simulink model "CaseD"  (R2016b)
settings: Solver=FixedStepAuto  StartTime=0.0  StopTime=time  FixedStep=dt  RelTol=1e-3
values from neighbouring files (symbols this model uses):
  C = [6; 0]    [main.m]
  dt = 0.01    [main.m]
  initial_eta = [1 0 0]'    [main.m]
  initial_eta_2 = [6 5 0]'    [main.m]
  initial_eta_4 = [7 0 0]'    [main.m]
  K_p = diag([0.2,0.2,0.1])    [main.m]
  mu = 0.1    [main.m]
  P_d = [2  0 ... (first row only)    [main.m]
  R = diag(r)    [main.m]
  r = [5; 3]    [main.m]
  U_max = 1    [main.m]
  U_ref = [(0:dt:time)' [zeros(floor(1*points/6),1) ... (first row only)    [main.m]
libraries: simulink x1
(part 1 of 2)
settings Model: Creator=helene  LastModifiedBy=kefin

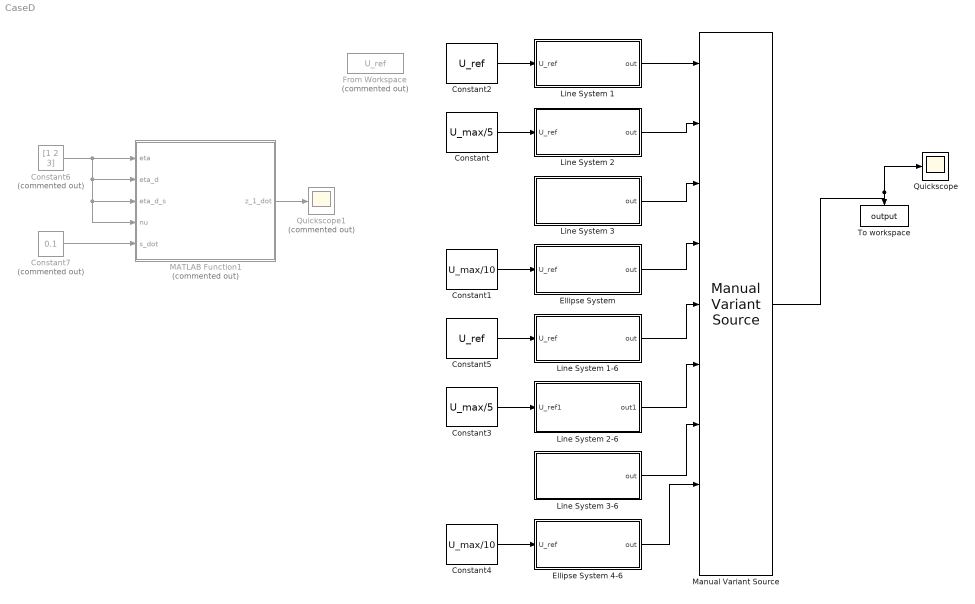
== system CaseD ==
  Constant : Constant  Value=U_max/5
  Constant1 : Constant  Value=U_max/10
  Constant2 : Constant  Value=U_ref
  Constant3 : Constant  Value=U_max/5
  Constant4 : Constant  Value=U_max/10
  Constant5 : Constant  Value=U_ref
  Constant6 : Constant  Commented=on  Value=[1 2 3]
  Constant7 : Constant  Commented=on  Value=0.1
  Ellipse System : Subsystem
  Ellipse System 4-6 : Subsystem
  From Workspace : FromWorkspace  Commented=on  VariableName=U_ref  SampleTime=dt
  Line System 1 : Subsystem
  Line System 1-6 : Subsystem
  Line System 2 : Subsystem
  Line System 2-6 : Subsystem
  Line System 3 : Subsystem
  Line System 3-6 : Subsystem
  MATLAB Function1 : MATLAB Function  Commented=on  TreatAsAtomicUnit=on
  Manual Variant Source : simulink/Signal Routing/Manual Variant Source  NumChoices=9  OverrideUsingVariant=V_8
  Quickscope : Scope
  Quickscope1 : Scope  Commented=on
  To workspace : ToWorkspace  VariableName=output  SampleTime=-1
      settings: StopFcn=plotting
  wires:
  Ellipse System/1(out) -> Manual Variant Source/4
  Manual Variant Source/1 -> Quickscope/1, To workspace/1
  Line System 1/1(out) -> Manual Variant Source/1
  Line System 2/1(out) -> Manual Variant Source/2
  Constant/1 -> Line System 2/1(U_ref)
  Line System 3/1(out) -> Manual Variant Source/3
  Constant1/1 -> Ellipse System/1(U_ref)
  Constant2/1 -> Line System 1/1(U_ref)
  Ellipse System 4-6/1(out) -> Manual Variant Source/8
  Line System 1-6/1(out) -> Manual Variant Source/5
  Line System 2-6/1(out1) -> Manual Variant Source/6
  Constant3/1 -> Line System 2-6/1(U_ref1)
  Line System 3-6/1(out) -> Manual Variant Source/7
  Constant4/1 -> Ellipse System 4-6/1(U_ref)
  Constant5/1 -> Line System 1-6/1(U_ref)
  Constant6/1 -> MATLAB Function1/4(nu), MATLAB Function1/3(eta_d_s), MATLAB Function1/2(eta_d), MATLAB Function1/1(eta)
  Constant7/1 -> MATLAB Function1/5(s_dot)
  MATLAB Function1/1(z_1_dot) -> Quickscope1/1

== system CaseD/Ellipse System ==
  U_ref : Inport
  Control law : Subsystem
  "Ellipse Mapper " : Subsystem
  Ellipse Speed Gauge : Subsystem
  Kinematic model : Subsystem
  Mux : Mux  Inputs=3
  Update Law : Subsystem
  out : Outport
  wires:
  U_ref/1 -> Ellipse Speed Gauge/1(U_ref)
  Update Law/1(s) -> Mux/3, Ellipse Speed Gauge/2(s), "Ellipse Mapper "/1(s)
  "Ellipse Mapper "/1(eta_d) -> Update Law/2(eta_d), Mux/2, Control law/4(eta_d)
  Kinematic model/1("eta ") -> Control law/1(eta), Update Law/4(eta), Mux/1
  Control law/1(nu) -> Kinematic model/1(nu)
  "Ellipse Mapper "/2(eta_d_s) -> Control law/3(eta_d_s), Update Law/3(eta_d_s)
  Ellipse Speed Gauge/1(U_s) -> Control law/2(U_s), Update Law/1(U_s)
  Mux/1 -> out/1

== system CaseD/Ellipse System 4-6 ==
  U_ref : Inport
  Control law1 : Subsystem
  "Ellipse Mapper " : Subsystem
  Ellipse Speed Gauge : Subsystem
  Kinematic model : Subsystem
  Mux : Mux  Inputs=3
  Update Law : Subsystem
  out : Outport
  wires:
  U_ref/1 -> Ellipse Speed Gauge/1(U_ref)
  Update Law/1(s) -> Ellipse Speed Gauge/2(s), "Ellipse Mapper "/1(s), Mux/3
  "Ellipse Mapper "/1(eta_d) -> Control law1/3(eta_d), Update Law/2(eta_d), Mux/2
  Kinematic model/1("eta ") -> Control law1/7(eta), Update Law/4(eta), Mux/1
  Control law1/1(new_nu) -> Control law1/8(nu), Kinematic model/1(nu)
  "Ellipse Mapper "/2(eta_d_s) -> Update Law/3(eta_d_s), Control law1/2(eta_d_s)
  Ellipse Speed Gauge/1(U_s) -> Control law1/1(U_s), Update Law/1(U_s)
  Mux/1 -> out/1
  Update Law/2(s_dot) -> Control law1/4(s_dot)
  Ellipse Speed Gauge/2(U_s_s) -> Control law1/5(U_s_s)
  "Ellipse Mapper "/3(eta_d_ss) -> Control law1/6(eta_d_ss)

== system CaseD/Line System 1 ==
  U_ref : Inport
  Control law : Subsystem
  Kinematic model : Subsystem
  Line Mapper : Subsystem
  Line Speed Gauge : Subsystem
  Mux : Mux  Inputs=3
  Update Law : Subsystem
  out : Outport
  wires:
  U_ref/1 -> Line Speed Gauge/1(U_ref)
  Update Law/1(s) -> Mux/3, Line Mapper/1("s ")
  Control law/1(nu) -> Kinematic model/1(nu)
  Line Mapper/2(eta_d_s) -> Control law/3(eta_d_s), Update Law/3(eta_d_s)
  Line Speed Gauge/1(U_s) -> Control law/2(U_s), Update Law/1(U_s)
  Line Mapper/1(eta_d) -> Control law/4(eta_d), Update Law/2(eta_d), Mux/2
  Kinematic model/1("eta ") -> Control law/1(eta), Update Law/4(eta), Mux/1
  Mux/1 -> out/1

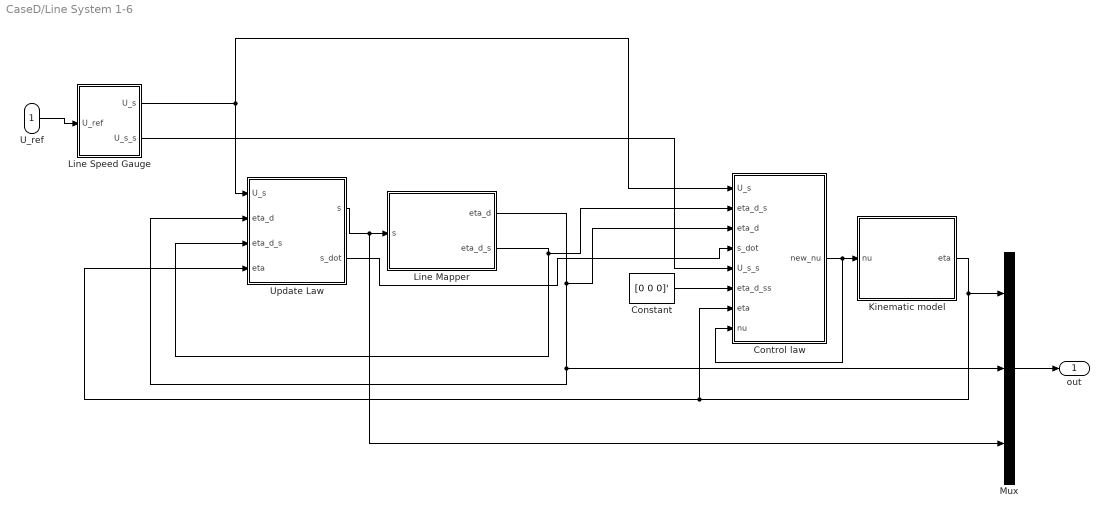
== system CaseD/Line System 1-6 ==
  U_ref : Inport
  Constant : Constant  Value=[0 0 0]'
  Control law : Subsystem
  Kinematic model : Subsystem
  Line Mapper : Subsystem
  Line Speed Gauge : Subsystem
  Mux : Mux  Inputs=3
  Update Law : Subsystem
  out : Outport
  wires:
  U_ref/1 -> Line Speed Gauge/1(U_ref)
  Update Law/1(s) -> Mux/3, Line Mapper/1("s ")
  Control law/1(new_nu) -> Control law/8(nu), Kinematic model/1(nu)
  Line Mapper/2(eta_d_s) -> Control law/2(eta_d_s), Update Law/3(eta_d_s)
  Line Speed Gauge/1(U_s) -> Control law/1(U_s), Update Law/1(U_s)
  Line Mapper/1(eta_d) -> Control law/3(eta_d), Update Law/2(eta_d), Mux/2
  Kinematic model/1("eta ") -> Control law/7(eta), Update Law/4(eta), Mux/1
  Mux/1 -> out/1
  Update Law/2(s_dot) -> Control law/4(s_dot)
  Line Speed Gauge/2(U_s_s) -> Control law/5(U_s_s)
  Constant/1 -> Control law/6(eta_d_ss)

== system CaseD/Line System 2 ==
  U_ref : Inport
  Control law : Subsystem
  Kinematic model : Subsystem
  Line Mapper : Subsystem
  Line Speed Gauge : Subsystem
  Mux : Mux  Inputs=3
  Update Law : Subsystem
  out : Outport
  wires:
  U_ref/1 -> Line Speed Gauge/1(U_ref)
  Update Law/1(s) -> Mux/3, Line Mapper/1("s ")
  Control law/1(nu) -> Kinematic model/1(nu)
  Line Mapper/2(eta_d_s) -> Update Law/3(eta_d_s), Control law/3(eta_d_s)
  Line Speed Gauge/1(U_s) -> Control law/2(U_s), Update Law/1(U_s)
  Line Mapper/1(eta_d) -> Update Law/2(eta_d), Mux/2, Control law/4(eta_d)
  Kinematic model/1("eta ") -> Control law/1(eta), Update Law/4(eta), Mux/1
  Mux/1 -> out/1

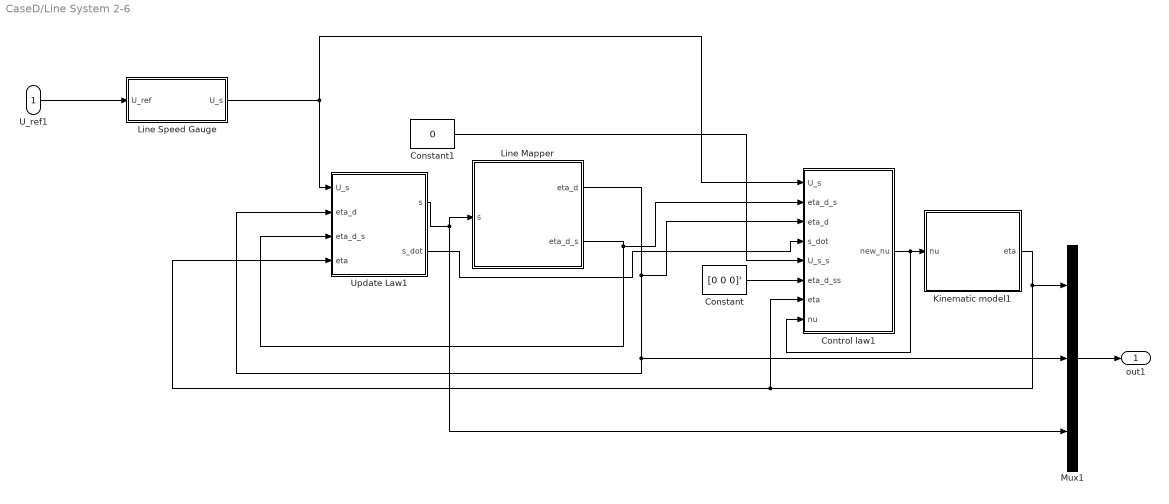
== system CaseD/Line System 2-6 ==
  U_ref1 : Inport
  Constant : Constant  Value=[0 0 0]'
  Constant1 : Constant  Value=0
  Control law1 : Subsystem
  Kinematic model1 : Subsystem
  Line Mapper : Subsystem
  Line Speed Gauge : Subsystem
  Mux1 : Mux  Inputs=3
  Update Law1 : Subsystem
  out1 : Outport
  wires:
  U_ref1/1 -> Line Speed Gauge/1(U_ref)
  Update Law1/1(s) -> Line Mapper/1("s "), Mux1/3
  Control law1/1(new_nu) -> Control law1/8(nu), Kinematic model1/1(nu)
  Line Mapper/2(eta_d_s) -> Control law1/2(eta_d_s), Update Law1/3(eta_d_s)
  Line Speed Gauge/1(U_s) -> Control law1/1(U_s), Update Law1/1(U_s)
  Line Mapper/1(eta_d) -> Control law1/3(eta_d), Update Law1/2(eta_d), Mux1/2
  Kinematic model1/1("eta ") -> Control law1/7(eta), Update Law1/4(eta), Mux1/1
  Mux1/1 -> out1/1
  Update Law1/2(s_dot) -> Control law1/4(s_dot)
  Constant1/1 -> Control law1/5(U_s_s)
  Constant/1 -> Control law1/6(eta_d_ss)

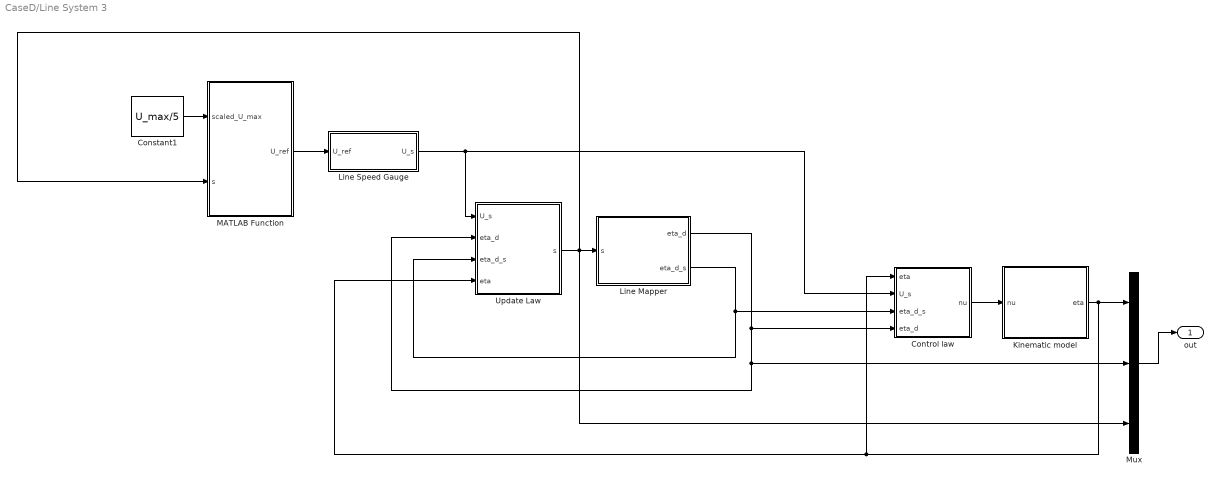
== system CaseD/Line System 3 ==
  Constant1 : Constant  Value=U_max/5
  Control law : Subsystem
  Kinematic model : Subsystem
  Line Mapper : Subsystem
  Line Speed Gauge : Subsystem
  MATLAB Function : MATLAB Function  TreatAsAtomicUnit=on
  Mux : Mux  Inputs=3
  Update Law : Subsystem
  out : Outport
  wires:
  Update Law/1(s) -> Line Mapper/1(s), Mux/3, MATLAB Function/2(s)
  Control law/1(nu) -> Kinematic model/1(nu)
  Line Mapper/2(eta_d_s) -> Control law/3(eta_d_s), Update Law/3(eta_d_s)
  Line Speed Gauge/1(U_s) -> Control law/2(U_s), Update Law/1(U_s)
  Line Mapper/1(eta_d) -> Control law/4(eta_d), Update Law/2(eta_d), Mux/2
  Kinematic model/1("eta ") -> Control law/1(eta), Update Law/4(eta), Mux/1
  Mux/1 -> out/1
  MATLAB Function/1(U_ref) -> Line Speed Gauge/1(U_ref)
  Constant1/1 -> MATLAB Function/1(scaled_U_max)

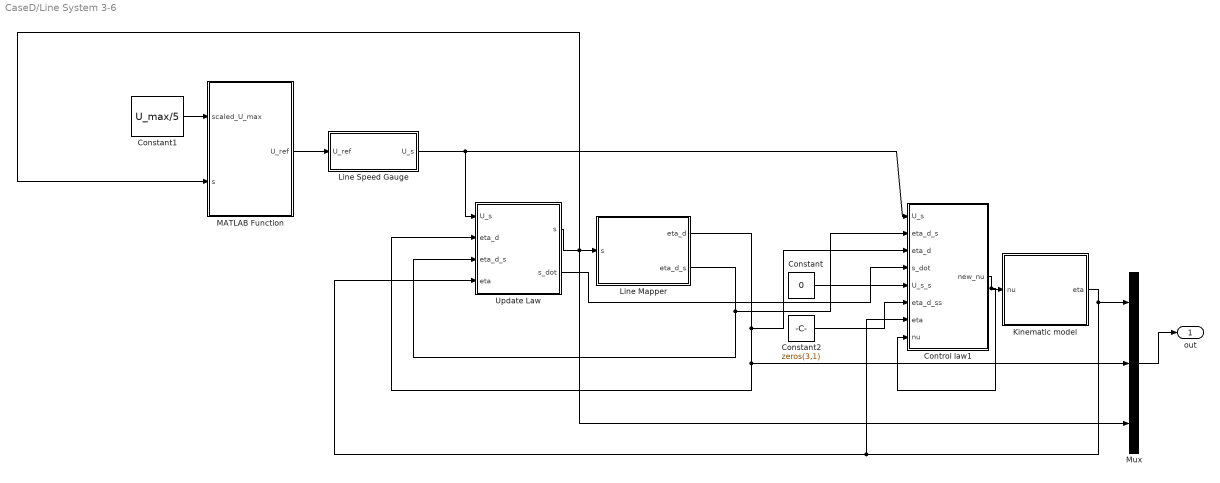
== system CaseD/Line System 3-6 ==
  Constant : Constant  Value=0
  Constant1 : Constant  Value=U_max/5
  Constant2 : Constant  Value=zeros(3,1)
  Control law1 : Subsystem
  Kinematic model : Subsystem
  Line Mapper : Subsystem
  Line Speed Gauge : Subsystem
  MATLAB Function : MATLAB Function  TreatAsAtomicUnit=on
  Mux : Mux  Inputs=3
  Update Law : Subsystem
  out : Outport
  wires:
  Update Law/1(s) -> Line Mapper/1(s), Mux/3, MATLAB Function/2(s)
  Control law1/1(new_nu) -> Control law1/8(nu), Kinematic model/1(nu)
  Line Mapper/2(eta_d_s) -> Control law1/2(eta_d_s), Update Law/3(eta_d_s)
  Line Speed Gauge/1(U_s) -> Control law1/1(U_s), Update Law/1(U_s)
  Line Mapper/1(eta_d) -> Control law1/3(eta_d), Update Law/2(eta_d), Mux/2
  Kinematic model/1("eta ") -> Control law1/7(eta), Update Law/4(eta), Mux/1
  Mux/1 -> out/1
  MATLAB Function/1(U_ref) -> Line Speed Gauge/1(U_ref)
  Constant1/1 -> MATLAB Function/1(scaled_U_max)
  Update Law/2(s_dot) -> Control law1/4(s_dot)
  Constant/1 -> Control law1/5(U_s_s)
  Constant2/1 -> Control law1/6(eta_d_ss)

== system CaseD/Ellipse System/Control law ==
  eta : Inport
  U_s : Inport  Port=2
  eta_d_s : Inport  Port=3
  eta_d : Inport  Port=4
  Control Law : MATLAB Function  TreatAsAtomicUnit=on
  K_p : Constant  Value=K_p
  Scope : Scope
  nu : Outport
  wires:
  K_p/1 -> Control Law/1(K_p)
  Control Law/1(nu) -> nu/1
  eta_d_s/1 -> Control Law/4(eta_d_s)
  U_s/1 -> Control Law/5(U_s)
  eta_d/1 -> Control Law/3(eta_d)
  eta/1 -> Control Law/2(eta)
  Control Law/2(z_1) -> Scope/1

== system CaseD/Ellipse System/Ellipse Mapper  ==
  s : Inport
  Constant : Constant  Value=R
  Constant1 : Constant  Value=C
  Ellipse Mapper : MATLAB Function  TreatAsAtomicUnit=on
  eta_d : Outport  PortDimensions=3
  eta_d_s : Outport  Port=2  PortDimensions=3
  wires:
  Ellipse Mapper/1(eta_d) -> eta_d/1
  Ellipse Mapper/2(eta_d_s) -> eta_d_s/1
  Constant1/1 -> Ellipse Mapper/2(C)
  Constant/1 -> Ellipse Mapper/3(R)
  s/1 -> Ellipse Mapper/1(s)

== system CaseD/Ellipse System/Ellipse Speed Gauge ==
  U_ref : Inport
  s : Inport  Port=2
  Constant : Constant  Value=r
  Ellipse : MATLAB Function  TreatAsAtomicUnit=on
  U_s : Outport
  wires:
  U_ref/1 -> Ellipse/1(U_ref)
  Ellipse/1(U_s) -> U_s/1
  Constant/1 -> Ellipse/3(r)
  s/1 -> Ellipse/2(s)

== system CaseD/Ellipse System/Kinematic model ==
  nu : Inport
  Integrator : Integrator  InitialCondition=initial_eta_4
  MATLAB Function : MATLAB Function  TreatAsAtomicUnit=on
  Product : Product  Multiplication=Matrix(*)
  Rotation matrix : MATLAB Function  TreatAsAtomicUnit=on
  Selector : Selector  InputPortWidth=3  IndexOptions=Starting index (dialog)  Indices=3  OutputSizes=1
  "eta " : Outport
  wires:
  Product/1 -> Integrator/1  "eta_dot"
  Integrator/1 -> MATLAB Function/1("eta "), Selector/1  "eta"
  nu/1 -> Product/2
  Rotation matrix/1(R) -> Product/1
  Selector/1 -> Rotation matrix/1(psi)
  MATLAB Function/1(eta) -> "eta "/1

== system CaseD/Ellipse System/Update Law ==
  U_s : Inport
  eta_d : Inport  Port=2
  eta_d_s : Inport  Port=3
  eta : Inport  Port=4
  Constant : Constant  Value=mu
  Integrator : Integrator
  Saturation : Saturate  UpperLimit=inf  LowerLimit=0
  Update Law : MATLAB Function  TreatAsAtomicUnit=on
  s : Outport
  wires:
  U_s/1 -> Update Law/1(U_s)
  Constant/1 -> Update Law/2(mu)
  eta_d_s/1 -> Update Law/3(eta_d_s)
  eta_d/1 -> Update Law/4(eta_d)
  Integrator/1 -> s/1
  eta/1 -> Update Law/5(eta)
  Saturation/1 -> Integrator/1
  Update Law/1(s_dot) -> Saturation/1

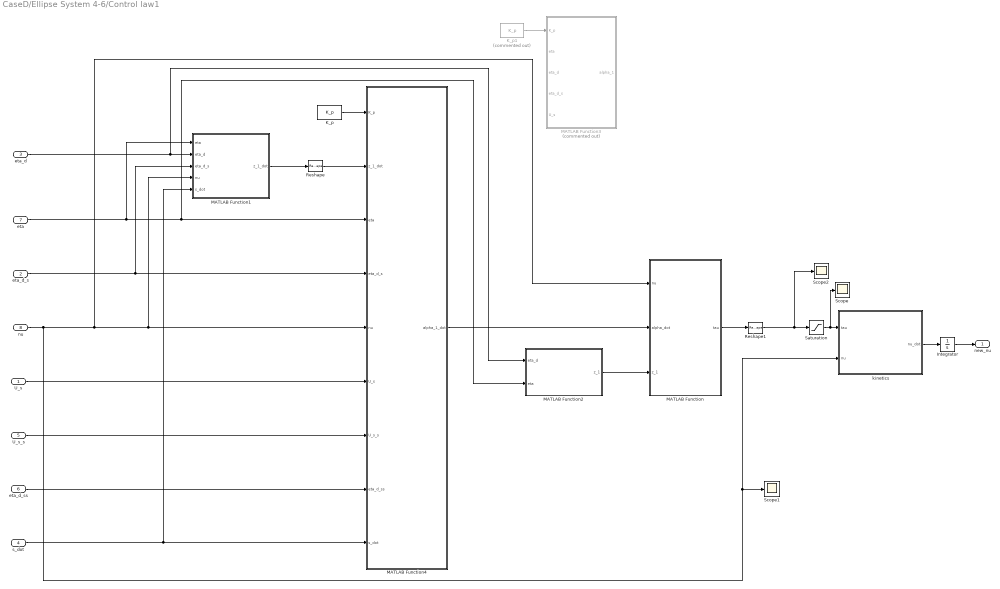
== system CaseD/Ellipse System 4-6/Control law1 ==
  U_s : Inport
  eta_d_s : Inport  Port=2
  eta_d : Inport  Port=3
  s_dot : Inport  Port=4
  U_s_s : Inport  Port=5
  eta_d_ss : Inport  Port=6
  eta : Inport  Port=7
  nu : Inport  Port=8
  Integrator : Integrator  InitialCondition=[0 0 0]'
  K_p : Constant  Value=K_p
  K_p1 : Constant  Commented=on  Value=K_p
  MATLAB Function : MATLAB Function  TreatAsAtomicUnit=on
  MATLAB Function1 : MATLAB Function  TreatAsAtomicUnit=on
  MATLAB Function2 : MATLAB Function  TreatAsAtomicUnit=on
  MATLAB Function3 : MATLAB Function  Commented=on  TreatAsAtomicUnit=on
  MATLAB Function4 : MATLAB Function  TreatAsAtomicUnit=on
  Reshape : Reshape  OutputDimensionality=Customize  OutputDimensions=[3,1]
  Reshape1 : Reshape  OutputDimensionality=Customize  OutputDimensions=[3,1]
  Saturation : Saturate  UpperLimit=[1.03 2.5 0.98]'  LowerLimit=-[1.03 2.5 0.98]'
  Scope : Scope
  Scope1 : Scope
  Scope2 : Scope
  kinetics : MATLAB Function  TreatAsAtomicUnit=on
  new_nu : Outport
  wires:
  eta_d_s/1 -> MATLAB Function1/3(eta_d_s), MATLAB Function4/4(eta_d_s)
  U_s/1 -> MATLAB Function4/6(U_s)
  eta_d/1 -> MATLAB Function2/1(eta_d), MATLAB Function1/2(eta_d)
  eta/1 -> MATLAB Function1/1(eta), MATLAB Function2/2(eta), MATLAB Function4/3(eta)
  MATLAB Function/1(tau) -> Reshape1/1
  K_p1/1 -> MATLAB Function3/1(K_p)
  MATLAB Function4/1(alpha_1_dot) -> MATLAB Function/2(alpha_dot)
  MATLAB Function1/1(z_1_dot) -> Reshape/1
  K_p/1 -> MATLAB Function4/1(K_p)
  U_s_s/1 -> MATLAB Function4/7(U_s_s)
  eta_d_ss/1 -> MATLAB Function4/8(eta_d_ss)
  s_dot/1 -> MATLAB Function1/5(s_dot), MATLAB Function4/9(s_dot)
  MATLAB Function2/1(z_1) -> MATLAB Function/3(z_1)
  Integrator/1 -> new_nu/1
  kinetics/1(nu_dot) -> Integrator/1
  nu/1 -> Scope1/1, kinetics/2(nu), MATLAB Function/1(nu), MATLAB Function1/4(nu), MATLAB Function4/5(nu)
  Saturation/1 -> Scope/1, kinetics/1(tau)
  Reshape/1 -> MATLAB Function4/2(z_1_dot)
  Reshape1/1 -> Scope2/1, Saturation/1

== system CaseD/Ellipse System 4-6/Ellipse Mapper  ==
  s : Inport
  Constant : Constant  Value=R
  Constant1 : Constant  Value=C
  Ellipse Mapper : MATLAB Function  TreatAsAtomicUnit=on
  eta_d : Outport  PortDimensions=3
  eta_d_s : Outport  Port=2  PortDimensions=3
  eta_d_ss : Outport  Port=3  PortDimensions=3
  wires:
  Ellipse Mapper/1(eta_d) -> eta_d/1
  Ellipse Mapper/2(eta_d_s) -> eta_d_s/1
  Constant1/1 -> Ellipse Mapper/2(C)
  Constant/1 -> Ellipse Mapper/3(R)
  s/1 -> Ellipse Mapper/1(s)
  Ellipse Mapper/3(eta_d_ss) -> eta_d_ss/1

== system CaseD/Ellipse System 4-6/Ellipse Speed Gauge ==
  U_ref : Inport
  s : Inport  Port=2
  Constant : Constant  Value=r
  Ellipse : MATLAB Function  TreatAsAtomicUnit=on
  U_s : Outport
  U_s_s : Outport  Port=2
  wires:
  U_ref/1 -> Ellipse/1(U_ref)
  Ellipse/1(U_s) -> U_s/1
  Constant/1 -> Ellipse/3(r)
  s/1 -> Ellipse/2(s)
  Ellipse/2(U_s_s) -> U_s_s/1

== system CaseD/Ellipse System 4-6/Kinematic model ==
  nu : Inport
  Integrator : Integrator  InitialCondition=initial_eta_4
  MATLAB Function : MATLAB Function  TreatAsAtomicUnit=on
  Product : Product  Multiplication=Matrix(*)
  Rotation matrix : MATLAB Function  TreatAsAtomicUnit=on
  Selector : Selector  InputPortWidth=3  IndexOptions=Starting index (dialog)  Indices=3  OutputSizes=1
  "eta " : Outport
  wires:
  Product/1 -> Integrator/1  "eta_dot"
  Integrator/1 -> MATLAB Function/1("eta "), Selector/1  "eta"
  nu/1 -> Product/2
  Rotation matrix/1(R) -> Product/1
  Selector/1 -> Rotation matrix/1(psi)
  MATLAB Function/1(eta) -> "eta "/1

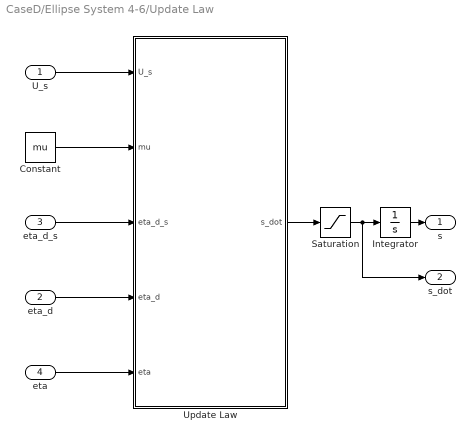
== system CaseD/Ellipse System 4-6/Update Law ==
  U_s : Inport
  eta_d : Inport  Port=2
  eta_d_s : Inport  Port=3
  eta : Inport  Port=4
  Constant : Constant  Value=mu
  Integrator : Integrator
  Saturation : Saturate  UpperLimit=inf  LowerLimit=0
  Update Law : MATLAB Function  TreatAsAtomicUnit=on
  s : Outport
  s_dot : Outport  Port=2
  wires:
  U_s/1 -> Update Law/1(U_s)
  Constant/1 -> Update Law/2(mu)
  eta_d_s/1 -> Update Law/3(eta_d_s)
  eta_d/1 -> Update Law/4(eta_d)
  Integrator/1 -> s/1
  eta/1 -> Update Law/5(eta)
  Saturation/1 -> s_dot/1, Integrator/1
  Update Law/1(s_dot) -> Saturation/1

== system CaseD/Line System 1/Control law ==
  eta : Inport
  U_s : Inport  Port=2
  eta_d_s : Inport  Port=3
  eta_d : Inport  Port=4
  Control Law : MATLAB Function  TreatAsAtomicUnit=on
  K_p : Constant  Value=K_p
  Scope : Scope
  nu : Outport
  wires:
  K_p/1 -> Control Law/1(K_p)
  Control Law/1(nu) -> nu/1
  eta_d_s/1 -> Control Law/4(eta_d_s)
  U_s/1 -> Control Law/5(U_s)
  eta_d/1 -> Control Law/3(eta_d)
  eta/1 -> Control Law/2(eta)
  Control Law/2(z_1) -> Scope/1

== system CaseD/Line System 1/Kinematic model ==
  nu : Inport
  Integrator : Integrator  InitialCondition=initial_eta
  Product : Product  Multiplication=Matrix(*)
  Rotation matrix : MATLAB Function  TreatAsAtomicUnit=on
  Selector : Selector  InputPortWidth=3  IndexOptions=Starting index (dialog)  Indices=3  OutputSizes=1
  "eta " : Outport
  wires:
  Product/1 -> Integrator/1  "eta_dot"
  Integrator/1 -> Selector/1, "eta "/1  "eta"
  nu/1 -> Product/2
  Rotation matrix/1(R) -> Product/1
  Selector/1 -> Rotation matrix/1(psi)

== system CaseD/Line System 1/Line Mapper ==
  "s " : Inport
  MATLAB Function : MATLAB Function  TreatAsAtomicUnit=on
  P_d : Constant  Value=P_d
  eta_d : Outport  PortDimensions=3
  eta_d_s : Outport  Port=2  PortDimensions=3
  wires:
  MATLAB Function/1(eta_d) -> eta_d/1
  MATLAB Function/2(eta_d_s) -> eta_d_s/1
  "s "/1 -> MATLAB Function/1(s)
  P_d/1 -> MATLAB Function/2(P_d)

== system CaseD/Line System 1/Line Speed Gauge ==
  U_ref : Inport
  Constant : Constant  Value=P_d
  Line : MATLAB Function  TreatAsAtomicUnit=on
  U_s : Outport
  wires:
  U_ref/1 -> Line/1(U_ref)
  Line/1(U_s) -> U_s/1
  Constant/1 -> Line/2(P_d)

== system CaseD/Line System 1/Update Law ==
  U_s : Inport
  eta_d : Inport  Port=2
  eta_d_s : Inport  Port=3
  eta : Inport  Port=4
  Constant : Constant  Value=mu
  Integrator : Integrator  LimitOutput=on  UpperSaturationLimit=1  LowerSaturationLimit=0
  Update Law : MATLAB Function  TreatAsAtomicUnit=on
  s : Outport
  wires:
  U_s/1 -> Update Law/1(U_s)
  Constant/1 -> Update Law/2(mu)
  eta_d_s/1 -> Update Law/3(eta_d_s)
  eta_d/1 -> Update Law/4(eta_d)
  Update Law/1(s_dot) -> Integrator/1
  Integrator/1 -> s/1
  eta/1 -> Update Law/5(eta)

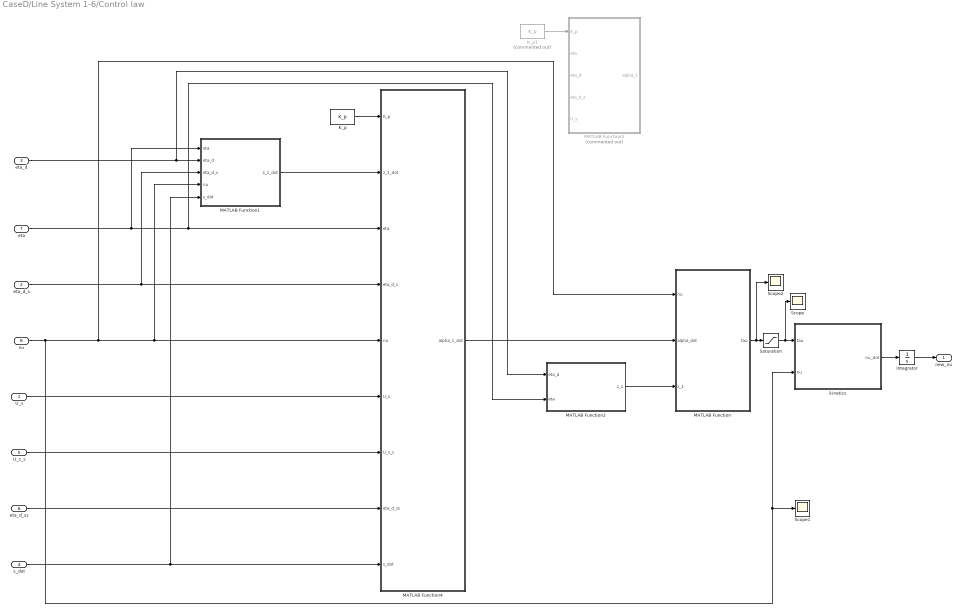
== system CaseD/Line System 1-6/Control law ==
  U_s : Inport
  eta_d_s : Inport  Port=2
  eta_d : Inport  Port=3
  s_dot : Inport  Port=4
  U_s_s : Inport  Port=5
  eta_d_ss : Inport  Port=6
  eta : Inport  Port=7
  nu : Inport  Port=8
  Integrator : Integrator  InitialCondition=[0 0 0]'
  K_p : Constant  Value=K_p
  K_p1 : Constant  Commented=on  Value=K_p
  MATLAB Function : MATLAB Function  TreatAsAtomicUnit=on
  MATLAB Function1 : MATLAB Function  TreatAsAtomicUnit=on
  MATLAB Function2 : MATLAB Function  TreatAsAtomicUnit=on
  MATLAB Function3 : MATLAB Function  Commented=on  TreatAsAtomicUnit=on
  MATLAB Function4 : MATLAB Function  TreatAsAtomicUnit=on
  Saturation : Saturate  UpperLimit=[1.03 2.5 0.98]'  LowerLimit=-[1.03 2.5 0.98]'
  Scope : Scope
  Scope1 : Scope
  Scope2 : Scope
  kinetics : MATLAB Function  TreatAsAtomicUnit=on
  new_nu : Outport
  wires:
  eta_d_s/1 -> MATLAB Function1/3(eta_d_s), MATLAB Function4/4(eta_d_s)
  U_s/1 -> MATLAB Function4/6(U_s)
  eta_d/1 -> MATLAB Function2/1(eta_d), MATLAB Function1/2(eta_d)
  eta/1 -> MATLAB Function1/1(eta), MATLAB Function2/2(eta), MATLAB Function4/3(eta)
  MATLAB Function/1(tau) -> Scope2/1, Saturation/1
  K_p1/1 -> MATLAB Function3/1(K_p)
  MATLAB Function4/1(alpha_1_dot) -> MATLAB Function/2(alpha_dot)
  MATLAB Function1/1(z_1_dot) -> MATLAB Function4/2(z_1_dot)
  K_p/1 -> MATLAB Function4/1(K_p)
  U_s_s/1 -> MATLAB Function4/7(U_s_s)
  eta_d_ss/1 -> MATLAB Function4/8(eta_d_ss)
  s_dot/1 -> MATLAB Function1/5(s_dot), MATLAB Function4/9(s_dot)
  MATLAB Function2/1(z_1) -> MATLAB Function/3(z_1)
  Integrator/1 -> new_nu/1
  kinetics/1(nu_dot) -> Integrator/1
  nu/1 -> Scope1/1, kinetics/2(nu), MATLAB Function/1(nu), MATLAB Function1/4(nu), MATLAB Function4/5(nu)
  Saturation/1 -> Scope/1, kinetics/1(tau)

== system CaseD/Line System 1-6/Kinematic model ==
  nu : Inport
  Integrator : Integrator  InitialCondition=initial_eta
  Product : Product  Multiplication=Matrix(*)
  Rotation matrix : MATLAB Function  TreatAsAtomicUnit=on
  Selector : Selector  InputPortWidth=3  IndexOptions=Starting index (dialog)  Indices=3  OutputSizes=1
  "eta " : Outport
  wires:
  Product/1 -> Integrator/1  "eta_dot"
  Integrator/1 -> Selector/1, "eta "/1  "eta"
  nu/1 -> Product/2
  Rotation matrix/1(R) -> Product/1
  Selector/1 -> Rotation matrix/1(psi)

== system CaseD/Line System 1-6/Line Mapper ==
  "s " : Inport
  MATLAB Function : MATLAB Function  TreatAsAtomicUnit=on
  P_d : Constant  Value=P_d
  eta_d : Outport  PortDimensions=3
  eta_d_s : Outport  Port=2  PortDimensions=3
  wires:
  MATLAB Function/1(eta_d) -> eta_d/1
  MATLAB Function/2(eta_d_s) -> eta_d_s/1
  "s "/1 -> MATLAB Function/1(s)
  P_d/1 -> MATLAB Function/2(P_d)

== system CaseD/Line System 1-6/Line Speed Gauge ==
  U_ref : Inport
  Constant : Constant  Value=P_d
  Line : MATLAB Function  TreatAsAtomicUnit=on
  U_s : Outport
  U_s_s : Outport  Port=2
  wires:
  U_ref/1 -> Line/1(U_ref)
  Line/1(U_s) -> U_s/1
  Constant/1 -> Line/2(P_d)
  Line/2(U_s_s) -> U_s_s/1

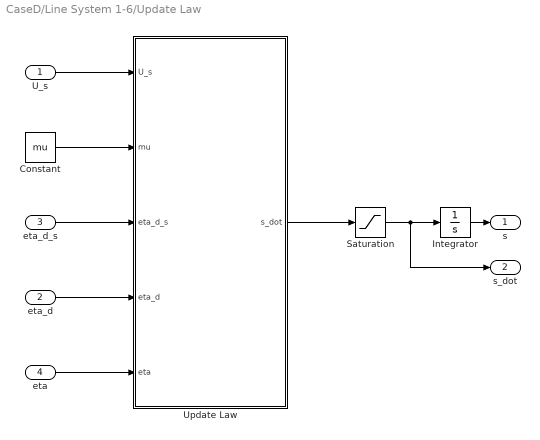
== system CaseD/Line System 1-6/Update Law ==
  U_s : Inport
  eta_d : Inport  Port=2
  eta_d_s : Inport  Port=3
  eta : Inport  Port=4
  Constant : Constant  Value=mu
  Integrator : Integrator  LimitOutput=on  UpperSaturationLimit=1  LowerSaturationLimit=0
  Saturation : Saturate  UpperLimit=inf  LowerLimit=0
  Update Law : MATLAB Function  TreatAsAtomicUnit=on
  s : Outport
  s_dot : Outport  Port=2
  wires:
  U_s/1 -> Update Law/1(U_s)
  Constant/1 -> Update Law/2(mu)
  eta_d_s/1 -> Update Law/3(eta_d_s)
  eta_d/1 -> Update Law/4(eta_d)
  Integrator/1 -> s/1
  eta/1 -> Update Law/5(eta)
  Update Law/1(s_dot) -> Saturation/1
  Saturation/1 -> s_dot/1, Integrator/1

== system CaseD/Line System 2/Control law ==
  eta : Inport
  U_s : Inport  Port=2
  eta_d_s : Inport  Port=3
  eta_d : Inport  Port=4
  Control Law : MATLAB Function  TreatAsAtomicUnit=on
  K_p : Constant  Value=K_p
  Scope : Scope
  nu : Outport
  wires:
  K_p/1 -> Control Law/1(K_p)
  Control Law/1(nu) -> nu/1
  eta_d_s/1 -> Control Law/4(eta_d_s)
  U_s/1 -> Control Law/5(U_s)
  eta_d/1 -> Control Law/3(eta_d)
  eta/1 -> Control Law/2(eta)
  Control Law/2(z_1) -> Scope/1

== system CaseD/Line System 2/Kinematic model ==
  nu : Inport
  Integrator : Integrator  InitialCondition=initial_eta_2
  Product : Product  Multiplication=Matrix(*)
  Rotation matrix : MATLAB Function  TreatAsAtomicUnit=on
  Selector : Selector  InputPortWidth=3  IndexOptions=Starting index (dialog)  Indices=3  OutputSizes=1
  "eta " : Outport
  wires:
  Product/1 -> Integrator/1  "eta_dot"
  Integrator/1 -> Selector/1, "eta "/1  "eta"
  nu/1 -> Product/2
  Rotation matrix/1(R) -> Product/1
  Selector/1 -> Rotation matrix/1(psi)

== system CaseD/Line System 2/Line Mapper ==
  "s " : Inport
  MATLAB Function : MATLAB Function  TreatAsAtomicUnit=on
  Memory : Memory
  P_d : Constant  Value=P_d
  eta_d : Outport  PortDimensions=3
  eta_d_s : Outport  Port=2  PortDimensions=3
  wires:
  MATLAB Function/1(eta_d) -> eta_d/1
  MATLAB Function/2(eta_d_s) -> eta_d_s/1
  "s "/1 -> MATLAB Function/1(s)
  P_d/1 -> MATLAB Function/2(P_d)
  Memory/1 -> MATLAB Function/3(s_proc_old)
  MATLAB Function/3(s_proc) -> Memory/1

== system CaseD/Line System 2/Line Speed Gauge ==
  U_ref : Inport
  Constant : Constant  Value=P_d
  Line : MATLAB Function  TreatAsAtomicUnit=on
  U_s : Outport
  wires:
  U_ref/1 -> Line/1(U_ref)
  Line/1(U_s) -> U_s/1
  Constant/1 -> Line/2(P_d)

== system CaseD/Line System 2/Update Law ==
  U_s : Inport
  eta_d : Inport  Port=2
  eta_d_s : Inport  Port=3
  eta : Inport  Port=4
  Constant : Constant  Value=mu
  Integrator : Integrator  UpperSaturationLimit=1  LowerSaturationLimit=0
  Update Law : MATLAB Function  TreatAsAtomicUnit=on
  s : Outport
  wires:
  U_s/1 -> Update Law/1(U_s)
  Constant/1 -> Update Law/2(mu)
  eta_d_s/1 -> Update Law/3(eta_d_s)
  eta_d/1 -> Update Law/4(eta_d)
  Integrator/1 -> s/1
  eta/1 -> Update Law/5(eta)
  Update Law/1(s_dot) -> Integrator/1

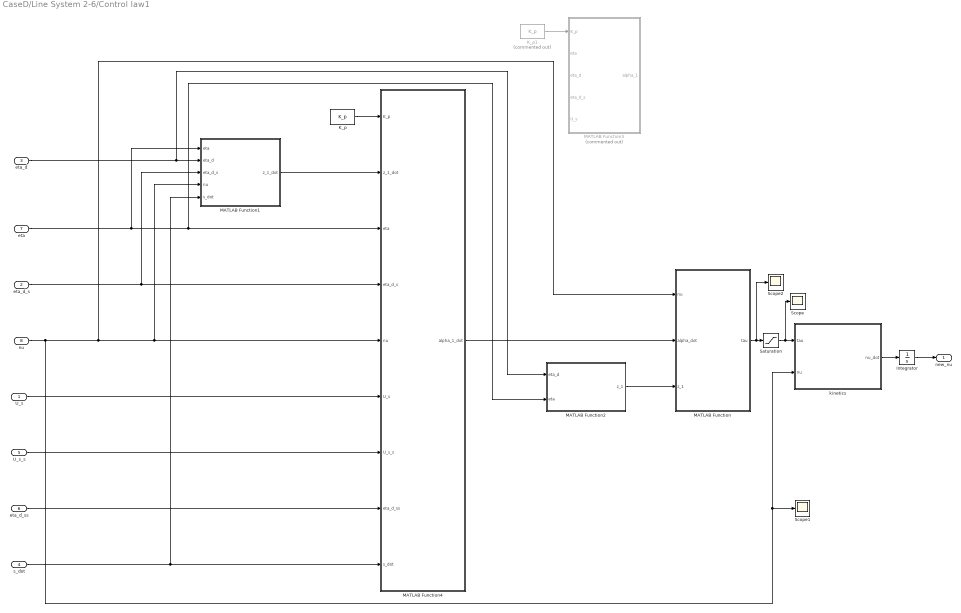
== system CaseD/Line System 2-6/Control law1 ==
  U_s : Inport
  eta_d_s : Inport  Port=2
  eta_d : Inport  Port=3
  s_dot : Inport  Port=4
  U_s_s : Inport  Port=5
  eta_d_ss : Inport  Port=6
  eta : Inport  Port=7
  nu : Inport  Port=8
  Integrator : Integrator  InitialCondition=[0 0 0]'
  K_p : Constant  Value=K_p
  K_p1 : Constant  Commented=on  Value=K_p
  MATLAB Function : MATLAB Function  TreatAsAtomicUnit=on
  MATLAB Function1 : MATLAB Function  TreatAsAtomicUnit=on
  MATLAB Function2 : MATLAB Function  TreatAsAtomicUnit=on
  MATLAB Function3 : MATLAB Function  Commented=on  TreatAsAtomicUnit=on
  MATLAB Function4 : MATLAB Function  TreatAsAtomicUnit=on
  Saturation : Saturate  UpperLimit=[1.03 2.5 0.98]'  LowerLimit=-[1.03 2.5 0.98]'
  Scope : Scope
  Scope1 : Scope
  Scope2 : Scope
  kinetics : MATLAB Function  TreatAsAtomicUnit=on
  new_nu : Outport
  wires:
  eta_d_s/1 -> MATLAB Function1/3(eta_d_s), MATLAB Function4/4(eta_d_s)
  U_s/1 -> MATLAB Function4/6(U_s)
  eta_d/1 -> MATLAB Function2/1(eta_d), MATLAB Function1/2(eta_d)
  eta/1 -> MATLAB Function1/1(eta), MATLAB Function2/2(eta), MATLAB Function4/3(eta)
  MATLAB Function/1(tau) -> Scope2/1, Saturation/1
  K_p1/1 -> MATLAB Function3/1(K_p)
  MATLAB Function4/1(alpha_1_dot) -> MATLAB Function/2(alpha_dot)
  MATLAB Function1/1(z_1_dot) -> MATLAB Function4/2(z_1_dot)
  K_p/1 -> MATLAB Function4/1(K_p)
  U_s_s/1 -> MATLAB Function4/7(U_s_s)
  eta_d_ss/1 -> MATLAB Function4/8(eta_d_ss)
  s_dot/1 -> MATLAB Function1/5(s_dot), MATLAB Function4/9(s_dot)
  MATLAB Function2/1(z_1) -> MATLAB Function/3(z_1)
  Integrator/1 -> new_nu/1
  kinetics/1(nu_dot) -> Integrator/1
  nu/1 -> Scope1/1, kinetics/2(nu), MATLAB Function/1(nu), MATLAB Function1/4(nu), MATLAB Function4/5(nu)
  Saturation/1 -> Scope/1, kinetics/1(tau)

== system CaseD/Line System 2-6/Kinematic model1 ==
  nu : Inport
  Integrator : Integrator  InitialCondition=initial_eta
  Product : Product  Multiplication=Matrix(*)
  Rotation matrix : MATLAB Function  TreatAsAtomicUnit=on
  Selector : Selector  InputPortWidth=3  IndexOptions=Starting index (dialog)  Indices=3  OutputSizes=1
  "eta " : Outport
  wires:
  Product/1 -> Integrator/1  "eta_dot"
  Integrator/1 -> Selector/1, "eta "/1  "eta"
  nu/1 -> Product/2
  Rotation matrix/1(R) -> Product/1
  Selector/1 -> Rotation matrix/1(psi)

== system CaseD/Line System 2-6/Line Mapper ==
  "s " : Inport
  MATLAB Function : MATLAB Function  TreatAsAtomicUnit=on
  Memory : Memory
  P_d : Constant  Value=P_d
  eta_d : Outport  PortDimensions=3
  eta_d_s : Outport  Port=2  PortDimensions=3
  wires:
  MATLAB Function/1(eta_d) -> eta_d/1
  MATLAB Function/2(eta_d_s) -> eta_d_s/1
  "s "/1 -> MATLAB Function/1(s)
  P_d/1 -> MATLAB Function/2(P_d)
  Memory/1 -> MATLAB Function/3(s_proc_old)
  MATLAB Function/3(s_proc) -> Memory/1

== system CaseD/Line System 2-6/Line Speed Gauge ==
  U_ref : Inport
  Constant : Constant  Value=P_d
  Line : MATLAB Function  TreatAsAtomicUnit=on
  U_s : Outport
  wires:
  U_ref/1 -> Line/1(U_ref)
  Line/1(U_s) -> U_s/1
  Constant/1 -> Line/2(P_d)

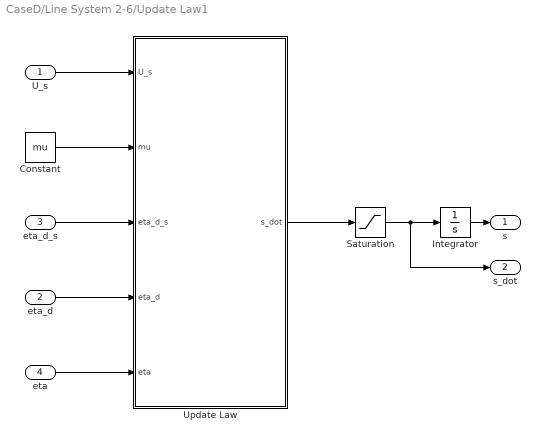
== system CaseD/Line System 2-6/Update Law1 ==
  U_s : Inport
  eta_d : Inport  Port=2
  eta_d_s : Inport  Port=3
  eta : Inport  Port=4
  Constant : Constant  Value=mu
  Integrator : Integrator  LimitOutput=on  UpperSaturationLimit=1  LowerSaturationLimit=0
  Saturation : Saturate  UpperLimit=inf  LowerLimit=0
  Update Law : MATLAB Function  TreatAsAtomicUnit=on
  s : Outport
  s_dot : Outport  Port=2
  wires:
  U_s/1 -> Update Law/1(U_s)
  Constant/1 -> Update Law/2(mu)
  eta_d_s/1 -> Update Law/3(eta_d_s)
  eta_d/1 -> Update Law/4(eta_d)
  Integrator/1 -> s/1
  eta/1 -> Update Law/5(eta)
  Update Law/1(s_dot) -> Saturation/1
  Saturation/1 -> s_dot/1, Integrator/1

== system CaseD/Line System 3/Control law ==
  eta : Inport
  U_s : Inport  Port=2
  eta_d_s : Inport  Port=3
  eta_d : Inport  Port=4
  Control Law : MATLAB Function  TreatAsAtomicUnit=on
  K_p : Constant  Value=K_p
  Scope : Scope
  nu : Outport
  wires:
  K_p/1 -> Control Law/1(K_p)
  Control Law/1(nu) -> nu/1
  eta_d_s/1 -> Control Law/4(eta_d_s)
  U_s/1 -> Control Law/5(U_s)
  eta_d/1 -> Control Law/3(eta_d)
  eta/1 -> Control Law/2(eta)
  Control Law/2(z_1) -> Scope/1

== system CaseD/Line System 3/Kinematic model ==
  nu : Inport
  Integrator : Integrator  InitialCondition=initial_eta_2
  Product : Product  Multiplication=Matrix(*)
  Rotation matrix : MATLAB Function  TreatAsAtomicUnit=on
  Selector : Selector  InputPortWidth=3  IndexOptions=Starting index (dialog)  Indices=3  OutputSizes=1
  "eta " : Outport
  wires:
  Product/1 -> Integrator/1  "eta_dot"
  Integrator/1 -> Selector/1, "eta "/1  "eta"
  nu/1 -> Product/2
  Rotation matrix/1(R) -> Product/1
  Selector/1 -> Rotation matrix/1(psi)

== system CaseD/Line System 3/Line Mapper ==
  s : Inport
  MATLAB Function : MATLAB Function  TreatAsAtomicUnit=on
  Memory : Memory
  P_d : Constant  Value=P_d
  eta_d : Outport  PortDimensions=3
  eta_d_s : Outport  Port=2  PortDimensions=3
  wires:
  MATLAB Function/1(eta_d) -> eta_d/1
  MATLAB Function/2(eta_d_s) -> eta_d_s/1
  s/1 -> MATLAB Function/1(s)
  P_d/1 -> MATLAB Function/3(P_d)
  Memory/1 -> MATLAB Function/2(s_proc_old)
  MATLAB Function/3(s_proc) -> Memory/1

== system CaseD/Line System 3/Line Speed Gauge ==
  U_ref : Inport
  Constant : Constant  Value=P_d
  Line : MATLAB Function  TreatAsAtomicUnit=on
  U_s : Outport
  wires:
  U_ref/1 -> Line/1(U_ref)
  Line/1(U_s) -> U_s/1
  Constant/1 -> Line/2(P_d)

== system CaseD/Line System 3/Update Law ==
  U_s : Inport
  eta_d : Inport  Port=2
  eta_d_s : Inport  Port=3
  eta : Inport  Port=4
  Constant : Constant  Value=mu
  Integrator : Integrator  UpperSaturationLimit=1  LowerSaturationLimit=0
  Update Law : MATLAB Function  TreatAsAtomicUnit=on
  s : Outport
  wires:
  U_s/1 -> Update Law/1(U_s)
  Constant/1 -> Update Law/2(mu)
  eta_d_s/1 -> Update Law/3(eta_d_s)
  eta_d/1 -> Update Law/4(eta_d)
  Update Law/1(s_dot) -> Integrator/1
  Integrator/1 -> s/1
  eta/1 -> Update Law/5(eta)

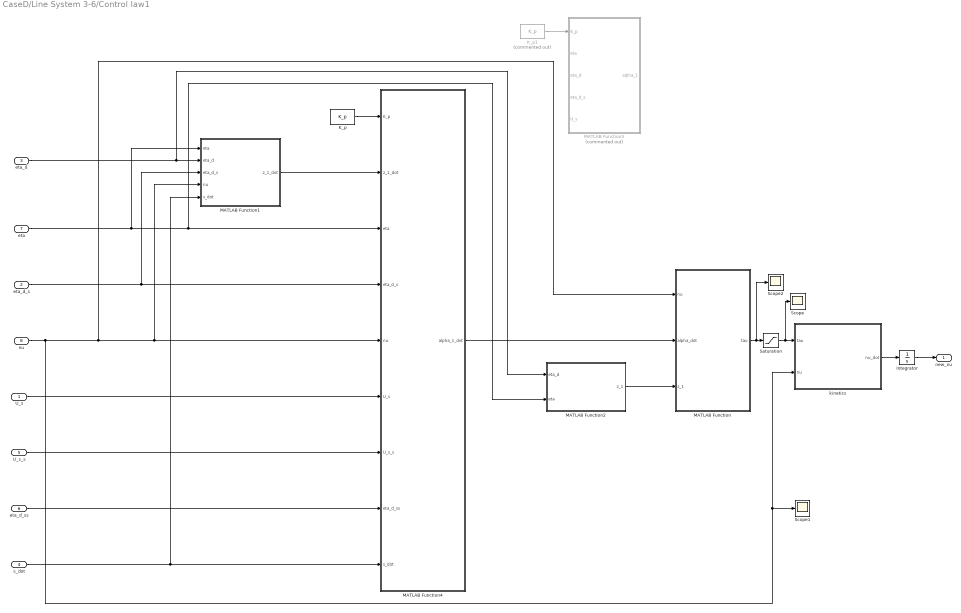
== system CaseD/Line System 3-6/Control law1 ==
  U_s : Inport
  eta_d_s : Inport  Port=2
  eta_d : Inport  Port=3
  s_dot : Inport  Port=4
  U_s_s : Inport  Port=5
  eta_d_ss : Inport  Port=6
  eta : Inport  Port=7
  nu : Inport  Port=8
  Integrator : Integrator  InitialCondition=[0 0 0]'
  K_p : Constant  Value=K_p
  K_p1 : Constant  Commented=on  Value=K_p
  MATLAB Function : MATLAB Function  TreatAsAtomicUnit=on
  MATLAB Function1 : MATLAB Function  TreatAsAtomicUnit=on
  MATLAB Function2 : MATLAB Function  TreatAsAtomicUnit=on
  MATLAB Function3 : MATLAB Function  Commented=on  TreatAsAtomicUnit=on
  MATLAB Function4 : MATLAB Function  TreatAsAtomicUnit=on
  Saturation : Saturate  UpperLimit=[1.03 2.5 0.98]'  LowerLimit=-[1.03 2.5 0.98]'
  Scope : Scope
  Scope1 : Scope
  Scope2 : Scope
  kinetics : MATLAB Function  TreatAsAtomicUnit=on
  new_nu : Outport
  wires:
  eta_d_s/1 -> MATLAB Function1/3(eta_d_s), MATLAB Function4/4(eta_d_s)
  U_s/1 -> MATLAB Function4/6(U_s)
  eta_d/1 -> MATLAB Function2/1(eta_d), MATLAB Function1/2(eta_d)
  eta/1 -> MATLAB Function1/1(eta), MATLAB Function2/2(eta), MATLAB Function4/3(eta)
  MATLAB Function/1(tau) -> Scope2/1, Saturation/1
  K_p1/1 -> MATLAB Function3/1(K_p)
  MATLAB Function4/1(alpha_1_dot) -> MATLAB Function/2(alpha_dot)
  K_p/1 -> MATLAB Function4/1(K_p)
  U_s_s/1 -> MATLAB Function4/7(U_s_s)
  eta_d_ss/1 -> MATLAB Function4/8(eta_d_ss)
  s_dot/1 -> MATLAB Function1/5(s_dot), MATLAB Function4/9(s_dot)
  MATLAB Function2/1(z_1) -> MATLAB Function/3(z_1)
  Integrator/1 -> new_nu/1
  kinetics/1(nu_dot) -> Integrator/1
  nu/1 -> Scope1/1, kinetics/2(nu), MATLAB Function/1(nu), MATLAB Function1/4(nu), MATLAB Function4/5(nu)
  Saturation/1 -> Scope/1, kinetics/1(tau)
  MATLAB Function1/1(z_1_dot) -> MATLAB Function4/2(z_1_dot)

== system CaseD/Line System 3-6/Kinematic model ==
  nu : Inport
  Integrator : Integrator  InitialCondition=initial_eta_2
  Product : Product  Multiplication=Matrix(*)
  Rotation matrix : MATLAB Function  TreatAsAtomicUnit=on
  Selector : Selector  InputPortWidth=3  IndexOptions=Starting index (dialog)  Indices=3  OutputSizes=1
  "eta " : Outport
  wires:
  Product/1 -> Integrator/1  "eta_dot"
  Integrator/1 -> Selector/1, "eta "/1  "eta"
  nu/1 -> Product/2
  Rotation matrix/1(R) -> Product/1
  Selector/1 -> Rotation matrix/1(psi)

== system CaseD/Line System 3-6/Line Mapper ==
  s : Inport
  MATLAB Function : MATLAB Function  TreatAsAtomicUnit=on
  Memory : Memory
  P_d : Constant  Value=P_d
  eta_d : Outport  PortDimensions=3
  eta_d_s : Outport  Port=2  PortDimensions=3
  wires:
  MATLAB Function/1(eta_d) -> eta_d/1
  MATLAB Function/2(eta_d_s) -> eta_d_s/1
  s/1 -> MATLAB Function/1(s)
  P_d/1 -> MATLAB Function/3(P_d)
  Memory/1 -> MATLAB Function/2(s_proc_old)
  MATLAB Function/3(s_proc) -> Memory/1

== system CaseD/Line System 3-6/Line Speed Gauge ==
  U_ref : Inport
  Constant : Constant  Value=P_d
  Line : MATLAB Function  TreatAsAtomicUnit=on
  U_s : Outport
  wires:
  U_ref/1 -> Line/1(U_ref)
  Line/1(U_s) -> U_s/1
  Constant/1 -> Line/2(P_d)

== system CaseD/Line System 3-6/Update Law ==
  U_s : Inport
  eta_d : Inport  Port=2
  eta_d_s : Inport  Port=3
  eta : Inport  Port=4
  Constant : Constant  Value=mu
  Integrator : Integrator  UpperSaturationLimit=1  LowerSaturationLimit=0
  Update Law : MATLAB Function  TreatAsAtomicUnit=on
  s : Outport
  s_dot : Outport  Port=2
  wires:
  U_s/1 -> Update Law/1(U_s)
  Constant/1 -> Update Law/2(mu)
  eta_d_s/1 -> Update Law/3(eta_d_s)
  eta_d/1 -> Update Law/4(eta_d)
  Update Law/1(s_dot) -> s_dot/1, Integrator/1
  Integrator/1 -> s/1
  eta/1 -> Update Law/5(eta)

== matlab function CaseD/Line System 3/Line Mapper/MATLAB Function ==
  data: s input; s_proc_old input; eta_d output; eta_d_s output; P_d input; s_proc output
function [eta_d, eta_d_s, s_proc] = linify(s, s_proc_old, P_d)
s = 1 - abs(mod(s, 2) - 1);
p_d = s.*[P_d(2, 1) - P_d(1, 1); P_d(2, 2) - P_d(1, 2)] + [P_d(1, 1); P_d(1, 2)];
psi_d = atan2(P_d(2, 2) - P_d(1, 2), P_d(2, 1) - P_d(1, 1));
if s_proc_old - s < 0
    psi_d = pi - psi_d;
end
p_d_s = [P_d(2, 1) - P_d(1, 1); P_d(2, 2) - P_d(1, 2)];
psi_d_s = 0;

eta_d = zeros(3, 1);
eta_d_s = zeros(3, 1);
eta_d = [p_d; psi_d];
eta_d_s = [p_d_s; psi_d_s];

s_proc = s;

== matlab function CaseD/Ellipse System/Kinematic model/MATLAB Function ==
  data: eta input; eta output
function eta = normalize(eta)
eta(3) = angdiff(0, eta(3));

== matlab function CaseD/Line System 3/Control law/Control Law ==
  data: K_p input; nu output; eta input; eta_d input; eta_d_s input; U_s input; z_1 output
function [nu, z_1] = control_law(K_p, eta, eta_d, eta_d_s, U_s)
psi = eta(3);
R = [cos(psi) -sin(psi) 0;
     sin(psi) cos(psi)  0;
     0        0         1];
 
 z_1_a = eta - eta_d;
% Here is where our eta_d would jump because of the parametrization.
% Instead of doing something hacky, we can redefine the control
% law such that it has the exact same gain.
% To compute the angular difference, we use angdiff:
z_1_psi = angdiff(eta_d(3), eta(3));
z_1_a(3) = z_1_psi;
z_1 = R'*z_1_a;
nu = -K_p*z_1 + R'*eta_d_s*U_s;

== matlab function CaseD/Line System 2/Control law/Control Law ==
  data: K_p input; nu output; eta input; eta_d input; eta_d_s input; U_s input; z_1 output
function [nu, z_1] = control_law(K_p, eta, eta_d, eta_d_s, U_s)
psi = eta(3);
R = [cos(psi) -sin(psi) 0;
     sin(psi) cos(psi)  0;
     0        0         1];
 
 z_1_a = eta - eta_d;
% Here is where our eta_d would jump because of the parametrization.
% Instead of doing something hacky, we can redefine the control
% law such that it has the exact same gain.
% To compute the angular difference, we use angdiff:
z_1_psi = angdiff(eta_d(3), eta(3));
z_1_a(3) = z_1_psi;
z_1 = R'*z_1_a;
nu = -K_p*z_1 + R'*eta_d_s*U_s;

== matlab function CaseD/Line System 1/Update Law/Update Law ==
  data: U_s input; s_dot output; mu input; eta_d_s input; eta_d input; eta input
function s_dot = update(U_s, mu, eta_d_s, eta_d, eta)
diff = eta - eta_d;
diff(3) = angdiff(eta_d(3), eta(3)); % Order is important here
s_dot = U_s - mu/norm(eta_d_s) * -diff' * eta_d_s;

== matlab function CaseD/Line System 1/Line Speed Gauge/Line ==
  data: U_ref input; U_s output; P_d input
function U_s = line(U_ref, P_d)
U_s = U_ref / sqrt(sum((P_d(:,2)-P_d(:,1)).^2));

== matlab function CaseD/Ellipse System/Control law/Control Law ==
  data: K_p input; nu output; eta input; eta_d input; eta_d_s input; U_s input; z_1 output
function [nu, z_1] = control_law(K_p, eta, eta_d, eta_d_s, U_s)
psi = eta(3);
R = [cos(psi) -sin(psi) 0;
     sin(psi) cos(psi)  0;
     0        0         1];
 
 z_1_a = eta - eta_d;
% Here is where our eta_d would jump because of the parametrization.
% Instead of doing something hacky, we can redefine the control
% law such that it has the exact same gain.
% To compute the angular difference, we use angdiff:
z_1_psi = angdiff(eta_d(3), eta(3));
z_1_a(3) = z_1_psi;
z_1 = R'*z_1_a;
nu = -K_p*z_1 + R'*eta_d_s*U_s;

== matlab function CaseD/Line System 1/Kinematic model/Rotation matrix ==
  data: psi input; R output
function R = rotation(psi)
R = [cos(psi) -sin(psi) 0;
     sin(psi) cos(psi)  0;
     0        0         1];

== matlab function CaseD/Ellipse System/Kinematic model/Rotation matrix ==
  data: psi input; R output
function R = rotation(psi)
R = [cos(psi) -sin(psi) 0;
     sin(psi) cos(psi)  0;
     0        0         1];

== matlab function CaseD/Line System 1/Control law/Control Law ==
  data: K_p input; nu output; eta input; eta_d input; eta_d_s input; U_s input; z_1 output
function [nu, z_1] = control_law(K_p, eta, eta_d, eta_d_s, U_s)
psi = eta(3);
R = [cos(psi) -sin(psi) 0;
     sin(psi) cos(psi)  0;
     0        0         1];
 
 z_1_a = eta - eta_d;
% Here is where our eta_d would jump because of the parametrization.
% Instead of doing something hacky, we can redefine the control
% law such that it has the exact same gain.
% To compute the angular difference, we use angdiff:
z_1_psi = angdiff(eta_d(3), eta(3));
z_1_a(3) = z_1_psi;
z_1 = R'*z_1_a;
nu = -K_p*z_1 + R'*eta_d_s*U_s;
% a = nu - tau
% We will have to compute tau here when using the system together with the
% kinematics

== matlab function CaseD/Ellipse System/Ellipse Speed Gauge/Ellipse ==
  data: U_ref input; s input; U_s output; r input
function U_s = ellipse(U_ref, s, r)
U_s = U_ref / sqrt((r(1)*sin(s))^2 + (r(2)*cos(s))^2);

== matlab function CaseD/Ellipse System/Update Law/Update Law ==
  data: U_s input; s_dot output; mu input; eta_d_s input; eta_d input; eta input
function s_dot = update(U_s, mu, eta_d_s, eta_d, eta)
diff = eta - eta_d;
diff(3) = angdiff(eta_d(3), eta(3)); % Order is important here
s_dot = U_s - mu/norm(eta_d_s) * -diff' * eta_d_s;

== matlab function CaseD/MATLAB Function1 ==
  data: eta input; z_1_dot output; eta_d input; eta_d_s input; nu input; s_dot input
function z_1_dot = derive_z_1(eta, eta_d, eta_d_s, nu, s_dot)
r = nu(3);
S = [0 -r 0; r 0 0; 0 0 0];

psi = eta(3);
R = [cos(psi) -sin(psi) 0;
     sin(psi) cos(psi)  0;
     0        0         1];
 
 z_1_a = eta - eta_d;
% Here is where our eta_d would jump because of the parametrization.
% Instead of doing something hacky, we can redefine the control
% law such that it has the exact same gain.
% To compute the angular difference, we use angdiff:
z_1_psi = angdiff(eta_d(3), eta(3));
z_1_a(3) = z_1_psi;
z_1 = R'*z_1_a;
z_1_dot = S'*z_1 + nu - R'*eta_d_s*s_dot;

== matlab function CaseD/Line System 1/Line Mapper/MATLAB Function ==
  data: s input; eta_d output; eta_d_s output; P_d input
function [eta_d, eta_d_s] = linify(s, P_d)
p_d = [P_d(2,1) - P_d(1,1); P_d(2,2) - P_d(1,2)]*s + [P_d(1,1); P_d(1,2)];
psi_d = atan2(P_d(2,2) - P_d(1,2), P_d(2,1) - P_d(1,1));

p_d_s = [P_d(2,1) - P_d(1,1); P_d(2,2) - P_d(1,2)];
psi_d_s = 0;

eta_d = [p_d; psi_d];
eta_d_s = [p_d_s; psi_d_s];

== matlab function CaseD/Ellipse System 4-6/Ellipse Mapper /Ellipse Mapper ==
  data: s input; eta_d output; C input; R input; eta_d_s output; eta_d_ss output
function [eta_d, eta_d_s, eta_d_ss] = ellipse(s, C, R)
rx = R(1,1);
ry = R(2,2);

eta_d = [rx*cos(s)+C(1);
         ry*sin(s)+C(2);
         %0;];
         atan2(ry*cos(s), -rx*sin(s))]; % + floor((s+2*pi-pi/2)/2/pi)*2*pi];

eta_d_s = [-rx*sin(s);
           ry*cos(s);
           %0;];
           rx*ry/(ry^2*cos(s)^2+rx^2*sin(s)^2)];
eta_d_ss = [-rx*cos(s);
            -ry*sin(s);
            -2*(rx^2*cos(s)*sin(s) - ry^2*cos(s)*sin(s))*rx*ry/(ry^2*cos(s)^2 + rx^2*sin(s)^2)^2];

== matlab function CaseD/Line System 2/Kinematic model/Rotation matrix ==
  data: psi input; R output
function R = rotation(psi)
R = [cos(psi) -sin(psi) 0;
     sin(psi) cos(psi)  0;
     0        0         1];

== matlab function CaseD/Line System 2/Line Mapper/MATLAB Function ==
  data: s input; P_d input; s_proc_old input; eta_d output; eta_d_s output; s_proc output
function [eta_d, eta_d_s, s_proc] = linify(s, P_d, s_proc_old)
s = 1 - abs(mod(s, 2) - 1);
p_d = s.*[P_d(2, 1) - P_d(1, 1); P_d(2, 2) - P_d(1, 2)] + [P_d(1, 1); P_d(1, 2)];
psi_d = atan2(P_d(2, 2) - P_d(1, 2), P_d(2, 1) - P_d(1, 1));
if s_proc_old - s < 0
    psi_d = pi - psi_d;
end
p_d_s = [P_d(2, 1) - P_d(1, 1); P_d(2, 2) - P_d(1, 2)];
psi_d_s = 0;

eta_d = zeros(3, 1);
eta_d_s = zeros(3, 1);
eta_d = [p_d; psi_d];
eta_d_s = [p_d_s; psi_d_s];

s_proc = s;

== matlab function CaseD/Line System 2/Line Speed Gauge/Line ==
  data: U_ref input; U_s output; P_d input
function U_s = line(U_ref, P_d)
U_s = U_ref / sqrt(sum((P_d(:,2)-P_d(:,1)).^2));

== matlab function CaseD/Line System 2/Update Law/Update Law ==
  data: U_s input; s_dot output; mu input; eta_d_s input; eta_d input; eta input
function s_dot = update(U_s, mu, eta_d_s, eta_d, eta)
s_dot = 0;
diff = eta - eta_d;
diff(3) = angdiff(eta_d(3), eta(3)); % Order is important here
s_dot = U_s - mu/norm(eta_d_s) * -abs(diff' * eta_d_s);

== matlab function CaseD/Line System 2-6/Control law1/MATLAB Function ==
  data: tau output; nu input; alpha_dot input; z_1 input
function tau = tau_function(nu, alpha_dot, z_1)
%% Parameters
% Rigid body and added mass
m = 14.79; 
I_z = 1.76; 
x_g = 0.0375; 
% y_g = 0.0;

X_u_dot = -2; 
Y_v_dot = -10; 
Y_r_dot = -0; 
N_r_dot = -1; 

% Max Values in Surge X, Sway Y and Yaw N
% X_max = 1.03; %[N]
% N_max = 2.50; %[N]
% Y_max = 0.98; %[N]

% Hydro surge, Hydro sway and Hydro Yaw Parameters
    % NB! We don't need most of them for now, that why they are commented
    % out, but don't remove them!!
X_u = -0.6555;  Y_v = -1.33;    N_v = 0.0; 
X_uu = 0.3545;  Y_vv = -2.776;  N_vv = -0.2088; 
X_uuu = -3.787; Y_vvv = -64.91; N_vvv = 0.0;
X_v = 0.0;      Y_r = -7.25;    N_r = -1.9; 
X_vv = -2.443;  Y_rr = -3.45;   N_rr = 0.75;
X_vvv = 0.0;    Y_rrr = 0.0;    N_rrr = 0.0;
                Y_rv = 0.805;   N_rv = 0.130;
                Y_vr = -0.845;  N_vr = 0.080;

%% Matrixes
u = nu(1); v = nu(2); r = nu(3); % I need a test values; 
    
a_11 = m-X_u_dot;   a_12 = 0;                   a_13 = 0; 
a_21 = 0;           a_22 = m-Y_v_dot ;          a_23 = m*x_g - Y_r_dot;
a_31 = 0;           a_32 = m*x_g - Y_r_dot;     a_33 = I_z - N_r_dot;

M = [a_11 a_12, a_13; a_12 a_22 a_23; a_31 a_32 a_33];

d_11_u =  -X_u - X_uu*abs(u) - X_uuu*u^2;
d_22_vr = -Y_v - Y_vv*abs(v) - Y_vvv*v^2   - Y_rv*abs(r);
d_23_vr = -Y_r - Y_vr*abs(v) - Y_rr*abs(r) - Y_rrr*r^2;
d_32_vr = -N_v - N_vv*abs(v) - N_vvv*v^2   - N_rv*abs(r);
d_33_vr = -N_r - N_vr*abs(v) - N_rr*abs(r) - N_rrr*r^2;

% The total damping matrix from the handbook page 53
D_tot = [d_11_u 0 0; 0 d_22_vr d_23_vr; 0 d_32_vr d_33_vr];

tau = D_tot*nu + M*alpha_dot - z_1;

== matlab function CaseD/Line System 3/Kinematic model/Rotation matrix ==
  data: psi input; R output
function R = rotation(psi)
R = [cos(psi) -sin(psi) 0;
     sin(psi) cos(psi)  0;
     0        0         1];

== matlab function CaseD/Ellipse System 4-6/Ellipse Speed Gauge/Ellipse ==
  data: U_ref input; s input; U_s output; r input; U_s_s output
function [U_s,U_s_s] = ellipse(U_ref, s, r)
U_s = U_ref / sqrt((r(1)*sin(s))^2 + (r(2)*cos(s))^2);
U_s_s = -(r(1)^2*cos(s)*sin(s) - r(2)^2*cos(s)*sin(s))*U_ref/(r(2)^2*cos(s)^2 + r(1)^2*sin(s)^2)^(3/2);

== matlab function CaseD/Line System 3/Line Speed Gauge/Line ==
  data: U_ref input; U_s output; P_d input
function U_s = line(U_ref, P_d)
U_s = U_ref / sqrt(sum((P_d(:,2)-P_d(:,1)).^2));

== matlab function CaseD/Line System 3/Update Law/Update Law ==
  data: U_s input; s_dot output; mu input; eta_d_s input; eta_d input; eta input
function s_dot = update(U_s, mu, eta_d_s, eta_d, eta)
s_dot = 0;
diff = eta - eta_d;
diff(3) = angdiff(eta_d(3), eta(3)); % Order is important here
s_dot = U_s - mu/norm(eta_d_s) * -diff' * eta_d_s;

== matlab function CaseD/Line System 3/MATLAB Function ==
  data: scaled_U_max input; U_ref output; s input
function U_ref = variable_s(scaled_U_max, s)
s = 1 - abs(mod(s, 2) - 1);
U_ref = scaled_U_max*(1.01 + sin(2*pi*s - pi/2));

== matlab function CaseD/Ellipse System/Ellipse Mapper /Ellipse Mapper ==
  data: s input; eta_d output; C input; R input; eta_d_s output
function [eta_d, eta_d_s] = ellipse(s, C, R)
rx = R(1,1);
ry = R(2,2);

eta_d = [rx*cos(s)+C(1);
         ry*sin(s)+C(2);
         %0;];
         atan2(ry*cos(s), -rx*sin(s))]; % + floor((s+2*pi-pi/2)/2/pi)*2*pi];

eta_d_s = [-rx*sin(s);
           ry*cos(s);
           %0;];
           rx*ry/(ry^2*cos(s)^2+rx^2*sin(s)^2)];

== matlab function CaseD/Ellipse System 4-6/Kinematic model/MATLAB Function ==
  data: eta input; eta output
function eta = normalize(eta)
eta(3) = angdiff(0, eta(3));

== matlab function CaseD/Ellipse System 4-6/Kinematic model/Rotation matrix ==
  data: psi input; R output
function R = rotation(psi)
R = [cos(psi) -sin(psi) 0;
     sin(psi) cos(psi)  0;
     0        0         1];

== matlab function CaseD/Ellipse System 4-6/Update Law/Update Law ==
  data: U_s input; s_dot output; mu input; eta_d_s input; eta_d input; eta input
function s_dot = update(U_s, mu, eta_d_s, eta_d, eta)
diff = eta - eta_d;
diff(3) = angdiff(eta_d(3), eta(3)); % Order is important here
s_dot = U_s - mu/norm(eta_d_s) * -diff' * eta_d_s;

== matlab function CaseD/Line System 2-6/Control law1/MATLAB Function1 ==
  data: eta input; z_1_dot output; eta_d input; eta_d_s input; nu input; s_dot input
function z_1_dot = derive_z_1(eta, eta_d, eta_d_s, nu, s_dot)
r = nu(3);
S = [0 -r 0; r 0 0; 0 0 0];

psi = eta(3);
R = [cos(psi) -sin(psi) 0;
     sin(psi) cos(psi)  0;
     0        0         1];
 
 z_1_a = eta - eta_d;
% Here is where our eta_d would jump because of the parametrization.
% Instead of doing something hacky, we can redefine the control
% law such that it has the exact same gain.
% To compute the angular difference, we use angdiff:
z_1_psi = angdiff(eta_d(3), eta(3));
z_1_a(3) = z_1_psi;
z_1 = R'*z_1_a;
z_1_dot = S'*z_1 + nu - R'*eta_d_s*s_dot;

== matlab function CaseD/Line System 1-6/Control law/kinetics ==
  data: tau input; nu_dot output; nu input
function nu_dot = CSE1_nu_dot(tau,nu)

u   = nu(1);
v   = nu(2);
r   = nu(3);

tau = [tau(1);tau(2);tau(3)];
%% MATRICES

m    = 14.79;   I_z  =  1.7600;   x_g = 0.0375;       % x_g  =  0.0460; % Table B.1


%% Added mass
X_ud  =     -2.0;											% Table B.1
					Y_vd =     -1.0;	N_vd =    -0.0;		% Table B.1 guestimate
					Y_rd =      -0.0;	N_rd =    -1.0;		% Table B.1

%% Total mass matrix
m_11 = m-X_ud;
m_22 = m-Y_vd;
m_23 = m*x_g-Y_rd;
m_32 = m*x_g-N_vd;
m_33 = I_z-N_rd;

M    = [m_11 0    0
        0    m_22 m_23
        0    m_32 m_33];
	
%% Damping coefficients
% Comments at the end of the lines indicate the old values used.
X_u		= -0.6555;		X_v		= 0;
X_uu 	= 0.3545;		X_vv	= -2.443;
X_uuu 	= -3.787;		X_vvv	= 0;

						Y_v		= -1.33; 			Y_r		= -7.250; % Y_r
						Y_vv	= -2.776;			Y_rr	= -3.450; % Y_rr
						Y_vvv	= -64.91;			Y_rrr	= 0;
						
						Y_rv	= -0.805;			Y_vr	= -0.845; % Y_rv, Y_vr

						N_v		= 0;				N_r		= -1.900; % N_r
						N_vv	= -0.2088;			N_rr	= -0.750; % N_rr
						N_vvv	= 0;				N_rrr	= 0;
						
						N_rv	= 0.130;			N_vr	= 0.080; % N_rv, N_vr

%% Correolis matrix
c_13 = -(m-Y_vd)*v-(m*x_g-Y_rd)*r;
c_23 = (m-X_ud)*u;
C    = [0     0     c_13
        0     0     c_23
        -c_13 -c_23 0   ];

%% Assembly of the damping matrix
d_11 = -X_u - X_uu*u - X_uuu*u^2;
d_22 = -Y_v - Y_vv*v - Y_vvv*v^2 - Y_rv*abs(r);
d_33 = -N_r - N_rr*abs(r) - N_rrr*r^2 - N_vr*abs(v); % using abs(r)

d_12 = -X_v - X_vv*v - X_vvv*v^2;
d_23 = -Y_r - Y_rr*abs(r) - Y_rrr*r^2 - Y_vr*abs(v);
d_32 = -N_v - N_vv*v - N_vvv*v^2 - N_rv*abs(r);

D    = [d_11 d_12 0
        0    d_22 d_23
        0    d_32 d_33];



%% CALCULATION
nu_dot = M\(tau-(C+D)*nu);

== matlab function CaseD/Line System 1-6/Kinematic model/Rotation matrix ==
  data: psi input; R output
function R = rotation(psi)
R = [cos(psi) -sin(psi) 0;
     sin(psi) cos(psi)  0;
     0        0         1];

== matlab function CaseD/Line System 1-6/Line Mapper/MATLAB Function ==
  data: s input; eta_d output; eta_d_s output; P_d input
function [eta_d, eta_d_s] = linify(s, P_d)
p_d = [P_d(2,1) - P_d(1,1); P_d(2,2) - P_d(1,2)]*s + [P_d(1,1); P_d(1,2)];
psi_d = atan2(P_d(2,2) - P_d(1,2), P_d(2,1) - P_d(1,1));

p_d_s = [P_d(2,1) - P_d(1,1); P_d(2,2) - P_d(1,2)];
psi_d_s = 0;

eta_d = [p_d; psi_d];
eta_d_s = [p_d_s; psi_d_s];

== matlab function CaseD/Line System 1-6/Line Speed Gauge/Line ==
  data: U_ref input; U_s output; P_d input; U_s_s output
function [U_s, U_s_s] = line(U_ref, P_d)
U_s = U_ref / sqrt(sum((P_d(:,2)-P_d(:,1)).^2));
U_s_s = 0;
